simulink model "ep4_6_3"  (R2018a)
settings: Solver=VariableStepAuto  StartTime=0.0  StopTime=1000  RelTol=1e-3
undefined symbols (not defined in the file or in its folder): Ki
libraries: simulink x1
settings Model: Creator=zheny  LastModifiedBy=zheny

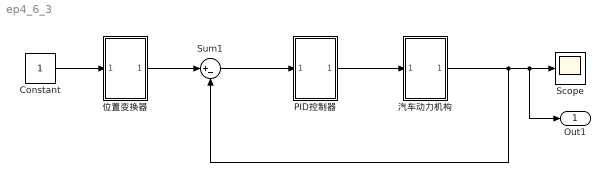
== system ep4_6_3 ==
  Constant : Constant
  PID控制器 : Subsystem  mask(PID控制器){Kp=1, Ki=Ki, Kd=0.01}
      mask help: y(n)=Kp*u(n)+Ki*x(n)+Kd*d(n)
      mask Help:
      | PID控制器
      | y(n)=Kp*u(n)+Ki*x(n)+Kd*d(n)
  Scope : Scope
  Sum1 : Sum  Inputs=|+-
  位置变换器 : Subsystem  mask(位置变换器){k=30, b=50}
      mask help: v=kx+b
      mask Help:
      | 位置变换器
      | v=kx+b
  汽车动力机构 : Subsystem  mask(汽车动力机构){m=1500, b=23}
      mask help: F=ma+bv
      mask Help:
      | 汽车动力机构
      | F=ma+bv
  Out1 : Outport
  wires:
  Constant/1 -> 位置变换器/1(In1)
  位置变换器/1(Out1) -> Sum1/1
  Sum1/1 -> PID控制器/1(In1)
  PID控制器/1(Out1) -> 汽车动力机构/1(In1)
  汽车动力机构/1(Out1) -> Sum1/2, Out1/1, Scope/1

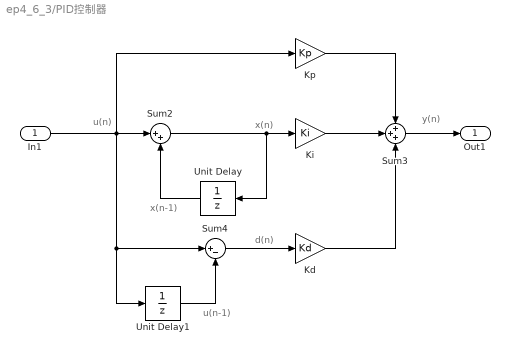
== system ep4_6_3/PID控制器 ==
  note: d(n)
  note: u(n-1)
  note: x(n-1)
  note: y(n)
  note: u(n)
  note: x(n)
  In1 : Inport
  Kd : Gain  Gain=Kd
  Ki : Gain  Gain=Ki
  Kp : Gain  Gain=Kp
  Sum2 : Sum  Inputs=|++
  Sum3 : Sum  Inputs=+++
  Sum4 : Sum  Inputs=|+-
  Unit Delay : UnitDelay  SampleTime=0.02
  Unit Delay1 : UnitDelay  SampleTime=0.02
  Out1 : Outport
  wires:
  Sum3/1 -> Out1/1
  Kp/1 -> Sum3/1
  Sum2/1 -> Unit Delay/1, Ki/1
  Sum4/1 -> Kd/1
  Unit Delay/1 -> Sum2/2
  In1/1 -> Sum4/1, Unit Delay1/1, Kp/1, Sum2/1
  Ki/1 -> Sum3/2
  Unit Delay1/1 -> Sum4/2
  Kd/1 -> Sum3/3

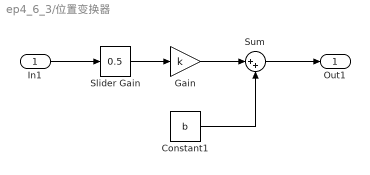
== system ep4_6_3/位置变换器 ==
  In1 : Inport
  Constant1 : Constant  Value=b
  Gain : Gain  Gain=k
  Slider Gain : simulink/Math Operations/Slider Gain  gain=0.5  low=0  high=1
  Sum : Sum  Inputs=|++
  Out1 : Outport
  wires:
  Constant1/1 -> Sum/2
  In1/1 -> Slider Gain/1
  Gain/1 -> Sum/1
  Slider Gain/1 -> Gain/1
  Sum/1 -> Out1/1

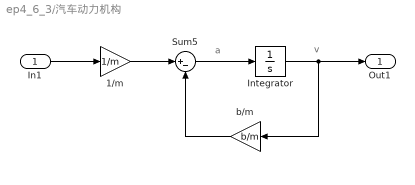
== system ep4_6_3/汽车动力机构 ==
  note: v
  note: a
  In1 : Inport
  1/m : Gain  Gain=1/m
  Integrator : Integrator
  Sum5 : Sum  Inputs=|+-
  b/m : Gain  Gain=b/m
  Out1 : Outport
  wires:
  Sum5/1 -> Integrator/1
  1/m/1 -> Sum5/1
  In1/1 -> 1/m/1
  Integrator/1 -> b/m/1, Out1/1
  b/m/1 -> Sum5/2
